simulink model "TwoCellImplementation"  (R2020a)
settings: Solver=VariableStepAuto  StartTime=0.0  StopTime=500  RelTol=1e-3
libraries: powerlib x12
settings Model: Creator=HP  LastModifiedBy=HP

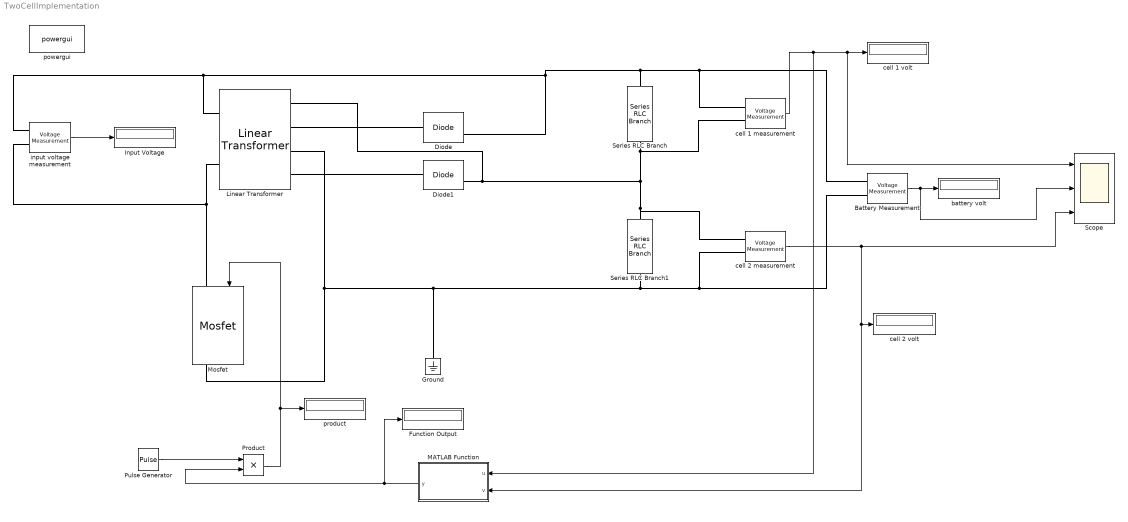
== system TwoCellImplementation ==
  "Battery Measurement " : powerlib/Measurements/Voltage Measurement  PhasorSimulation=off  OutputType=Complex  PSBequivalent=0
  Diode : powerlib/Power Electronics/Diode  Ron=0.001  Lon=0  Vf=0.8  IC=0  UseSnubber=0  Rs=500  Cs=250e-9  Measurements=on
  Diode1 : powerlib/Power Electronics/Diode  Ron=0.001  Lon=0  Vf=0.8  IC=0  UseSnubber=0  Rs=500  Cs=250e-9  Measurements=on
  Function Output : Display
  Ground : powerlib/Elements/Ground  LConnTagsString=a
  Input Voltage : Display
  Linear Transformer : powerlib/Elements/Linear Transformer  UNITS=SI  NominalPower=[100 55000]  winding1=[10 0.02 45e-6]  winding2=[5 0.02 288e-6]  ThreeWindings=on  winding3=[5 0.02 288e-6]  RmLm=[1.0805e+06 2866]  Measurements=None  DataType=on
  MATLAB Function : MATLAB Function  TreatAsAtomicUnit=on
  Mosfet : powerlib/Power Electronics/Mosfet  Ron=1.5  Lon=0  Rd=2  Vfd=0  IC=0  Rs=1500  Cs=288e-7  Measurements=on
  Product : Product
  Pulse Generator : DiscretePulseGenerator  PulseType=Time based  Period=10  PulseWidth=50
  Scope : Scope  NumInputPorts=3
  Series RLC Branch : powerlib/Elements/Series RLC Branch  LConnTagsString=__new0  RConnTagsString=__new0  BranchType=C  Resistance=1  Inductance=1e-3  SetiL0=off  InitialCurrent=0  Capacitance=5  Setx0=on  InitialVoltage=3  Measurements=None
  Series RLC Branch1 : powerlib/Elements/Series RLC Branch  LConnTagsString=__new0  RConnTagsString=__new0  BranchType=C  Resistance=1  Inductance=1e-3  SetiL0=off  InitialCurrent=0  Capacitance=5  Setx0=on  InitialVoltage=3.4  Measurements=None
  "battery volt " : Display
  "cell 1 measurement " : powerlib/Measurements/Voltage Measurement  PhasorSimulation=off  OutputType=Complex  PSBequivalent=0
  "cell 1 volt " : Display
  "cell 2 measurement " : powerlib/Measurements/Voltage Measurement  PhasorSimulation=off  OutputType=Complex  PSBequivalent=0
  "cell 2 volt " : Display
  "input voltage measurement " : powerlib/Measurements/Voltage Measurement  PhasorSimulation=off  OutputType=Complex  PSBequivalent=0
  powergui : powerlib/powergui  Priority=1  SimulationMode=Continuous  SampleTime=50e-6  frequency=60  Iterations=50  frequencyindice=0  Pbase=100e6  ErrMax=1e-4  UnitsV=kV  UnitsW=MW  buscounter=0  FunctionMessages=off  echomessages=off  EnableUseOfTLC=off  CurrentSourceSwitches=off  DisableSnubberDevices=off  DisableRonSwitches=off  DisableVfSwitches=off  DisplayEquations=off  AutomaticDiscreteSolvers=off  SolverType=Tustin/Backward Euler (TBE)  Interpol=off  ExternalGateDelay=off  methode=off  Ts=100  x0status=blocks  SPID=on  SwTol=0  HookPort=off  NonlinearTolerance=1e-4  nMaxIteration=100  ContinueOnMaxIteration=off  RestoreLinks=warning  ResistiveCurrentMeasurement=off  Frange=[0:2:500]  Ylog=off  Xlog=on  ShowGrid=off  save=off  variable=ZData  structure=0  ZoomFFT=off  StartTime=0.0  cycles=1  DisplayStyle=1  fundamental=60  FreqAxis=off  MaxFrequency=1000  frequencyindicesteady=1  RmsSteady=1  display=off
  "product " : Display
  wires:
  Pulse Generator/1 -> Product/1
  Product/1 -> Mosfet/1, "product "/1
  MATLAB Function/1(y) -> Function Output/1, Product/2
  "cell 1 measurement "/1 -> MATLAB Function/1(u), Scope/1, "cell 1 volt "/1
  "cell 2 measurement "/1 -> Scope/3, MATLAB Function/2(v), "cell 2 volt "/1
  "Battery Measurement "/1 -> Scope/2, "battery volt "/1
  "input voltage measurement "/1 -> Input Voltage/1
  connections:
  Linear Transformer/RConn2 -- Diode/LConn1
  Linear Transformer/RConn4 -- Diode1/LConn1
  Diode/RConn1 -- Linear Transformer/LConn1 -- "input voltage measurement "/LConn1 -- "Battery Measurement "/LConn1 -- "cell 1 measurement "/LConn1 -- Series RLC Branch/LConn1
  Series RLC Branch/RConn1 -- "cell 1 measurement "/LConn2 -- Linear Transformer/RConn1 -- Diode1/RConn1 -- "cell 2 measurement "/LConn1 -- Series RLC Branch1/LConn1
  Linear Transformer/LConn2 -- "input voltage measurement "/LConn2 -- Mosfet/LConn1
  Linear Transformer/RConn3 -- Mosfet/RConn1 -- "Battery Measurement "/LConn2 -- "cell 2 measurement "/LConn2 -- Series RLC Branch1/RConn1 -- Ground/LConn1

== matlab function TwoCellImplementation/MATLAB Function ==
  data: u input; y output; v input
function y = fcn(u,v)
if(u <= v && u >= v)
    y = 0;
else 
    y = 1;
end
